simulink model "b_microCHP_constant"  (Simulink 7.6)
settings: Solver=ode45  StartTime=0  StopTime=10000000  RelTol=1e-3
undefined symbols (not defined in the file): carmen
settings Model: Creator=Sebastian  LastModifiedBy=fabian.ille  SimulationMode=accelerator
settings OptimizationCC: InitFltsAndDblsToZero=on
settings DebuggingCC: StrictBusMsg=Warning
settings SFSimCC: SimParseCustomCode=off

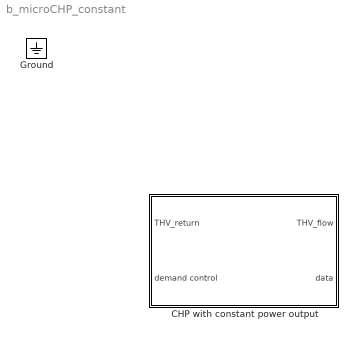
== system b_microCHP_constant ==
  CHP with constant power output : Subsystem  mask{P_th=11520, P_el=5500, P_fuel=22030, T_flow_setpoint=80, T_return_max=75}
      mask prompts: P_th "Nominal heating power [W] - at T_flow_out of 60°C"; P_el "Electrical power [W]"; P_fuel "Fuel power [W]"; T_flow_setpoint "T_flow_setpoint [°C] - Setpoint temperature of thermostat"; T_return_max "T_return_max [°C] - safety shutdown temperature"
      mask help:
      | This block is based on characteristic curves calculating heating capacity and representing a thermostat-controlled three-way mixer valve situated in the inlet flow of a gas driven micro-CHP called "Dachs" by Senertec. External mass flow rate, outlet flow temperature and heating power factor depend on inlet return temperature and are calculated by 1-D lookup-tables based on measured data.
      | The scaling is based on a heating power of 12.52 kW, an electrical power of 5.5 kW, a fuel power of 22,03 kW and a maximum external mass flow rate of 0.14 kg/s.
      | Mass flow rate and thermal inertia are linearly resized according to the inputed nominal heating power.
      mask Help: eval('filetest (''manual.htm#electric_heating'')')
      mask Display: plot(0,0,100,100,[50,50,60,40,50],[55,40,70,60,90],[59,50],[48,40])
  Ground : Ground  IOType=siggen

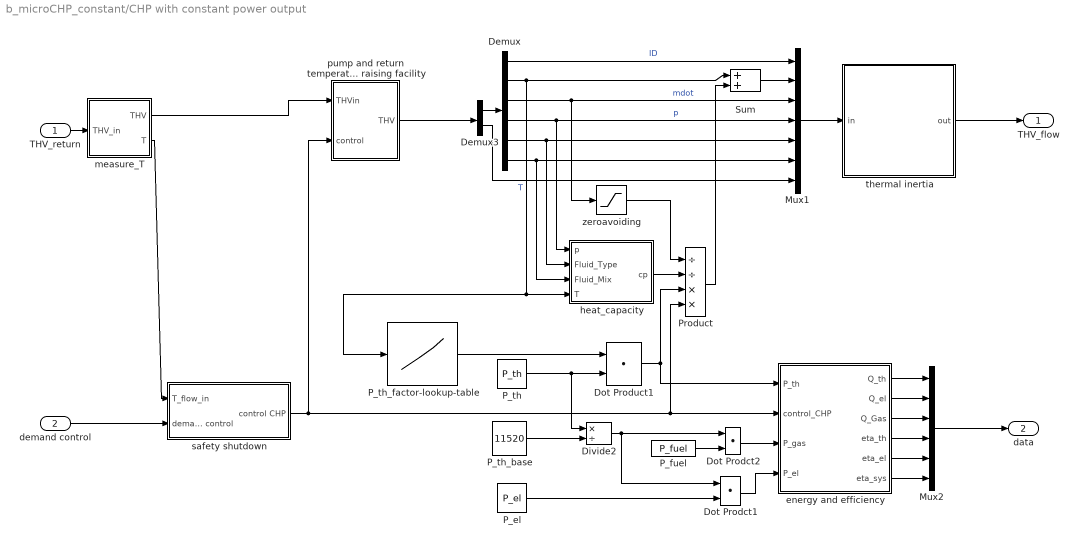
== system b_microCHP_constant/CHP with constant power output ==
  THV_return : Inport
  demand control : Inport  Port=2
  Demux : Demux  Outputs=[1 1 1 1 1 1]
  Demux3 : Demux  Outputs=[6 14]
  Divide2 : Product  Inputs=*/
  Dot Prodct1 : DotProduct  InputSameDT=on  OutDataTypeStr=Inherit: Inherit via internal rule
  Dot Prodct2 : DotProduct  InputSameDT=on  OutDataTypeStr=Inherit: Inherit via internal rule
  Dot Product1 : DotProduct  InputSameDT=on  OutDataTypeStr=Inherit: Inherit via internal rule
  Mux1 : Mux  Inputs=[1 1 1 1 1 1 14]
  Mux2 : Mux  Inputs=6
  P_el : Constant  Value=P_el
  P_fuel : Constant  Value=P_fuel
  P_th : Constant  Value=P_th
  P_th_base : Constant  Value=11520
  P_th_factor-lookup-table : Lookup_n-D  NumberOfTableDimensions=1  BreakpointsForDimension1=[45,50,60,65,74]  BreakpointsForDimension2=[44,80]  BreakpointsForDimension3=[1:2]  BreakpointsForDimension4=[1:2]  Table=[1.09 1.06 1 0.98 0.94]  InputSameDT=on
  Product : Product  Inputs=//**  SaturateOnIntegerOverflow=on  RndMeth=Zero  InputSameDT=on  OutDataTypeStr=Inherit: Same as first input
  Sum : Sum  SaturateOnIntegerOverflow=on  InputSameDT=on  OutDataTypeStr=Inherit: Same as first input
  energy and efficiency : Subsystem
  heat_capacity : Subsystem
      mask Type: heat capacity
      mask Description:
      | Calculates the  heat_capacity of fluids [J/(kg*K)].
      | Calls calls the function "hcap" in the CARNOT library "carlib".
      | Definition of the fluid types
      | fluid-ID  material           remarks on fluid mix
      | 1           water              vapourcontent in the 2-phase region
      | 2           air                   is (kg water) / (kg air)
      | 3           cotton oil
      | 4           silicone oil
      | 5           water-glycol    gives the volume partition [0..1] of glycol
      mask Help: eval('htmlhelp (''chap_4_2h.htm#heat_capacity'')')
  measure_T : Subsystem  mask(temperature measurement sensor){tc=10, t0=25}
      mask prompts: tc "time constant of sensor [s]"; t0 "initial temperature [degree centigrade]"
      mask help: Measurement sensor for temperatures with first-oder hold. Temperature is in degree centigrade.
      mask init:
      | tc = 1/max(tc, 0.001);
      mask Help: eval('man (''measure_T'')')
      mask Display: plot(-18,0,30,20,[0 20],[0 0],[10 10 8 8 12 12 10],[0 8 8 17 17 8 8],[10 10 9 9 11 11 10 9],[15 10 10 9 9 10 9 10])
  pump and return temperature raising facility : Subsystem  mask( Pump and return temperature raising facility){fluid_id=water, mix=0, dia=0.02, power=100, p0=3e5}
      mask prompts: fluid_id "fluid"; mix "percentage of fluid mix [0..1]"; dia "diameter at in- and outlet [m]"; power "electric power consumption [W]"; p0 "system pressure [Pa]"
      mask help:
      | In this modul a pump and a return temperature raising facility are modelled by two lookup-tables. They are based on measured data.
      |
      | The mass flow-lookup table gives out the mass flow (outside of CHP) depending on the return flow temperature T_return (outside of CHP). The return flow temperature (inside of CHP) is kept on 74°C by means of a thermostatic mixing valve.
      |
      | The T_flow-lookup table gives out the flow temperature T_flow depending on the return flow temperature (outside of CHP).
      |
      | The mass flow (outside of CHP) varies by means of multiplication with a factor f_flowSetpoint depending on the flow setpoint temperature T_flowSetpoint.
      | f_flowSetpoint is calculated according to the following formula:
      | (T_flow-T_return)/(T_flowSetpoint-T_return).
      |
      | The mass flow (outside of CHP) depends also on the nominal heating power P_heating and is therefor multiplied with a factor f_power.
      | f_power is calculated according to the following formula: P_heating/11520.
      mask init:
      | mix = min(1, max(0, mix));
      | dia = max(0.001, dia);
      | p0 = max(p0, 1e5);
      mask Help: eval('htmlhelp (''chap_4_2p.htm#pump_const'')')
      mask StyleString: popup(water|air|cotton_oil|silicone_oil|water_glycol_mix),edit,edit,edit,edit
      mask Display: plot(0,0,100,100,[40,70,40,30,30,40,60,70,70,60,40],[70,50,30,40,60,70,70,60,40,30,30])
  safety shutdown : Subsystem
      mask Type: control of safety shutdown
      mask Description:
      | CHP ON: T_return < T_return_max
      | CHP OFF: T_return > T_return_max
      mask Display: plot(-30,0,150,100,[70,100,40,10,70,70,10,10],[50,80,80,50,50,20,20,50],[100,70],[50,20],[20,50,50,20,20],[40,40,30,30,40],[62,62,62,61,59,58,58,60],[42,41,39,38,38,40,42,43],[61,62,62,61,60,59,58,58,58,59],[32,31,30,28,27,28,28,30,31,32])
  thermal inertia : Subsystem  LoadFcn=carmen('call');  mask(simple water storage){vol=0.00175*P_th/1000+ 0.0021, d=0.1, stand=standing cylinder, cond=1, uloss=1, tini=25, nodes=3, mpts=1, T_amb=15}
      mask prompts: vol "volume [m³]"; d "diameter [m]"; stand "position"; cond "axial heat conductivity [W/(m*K)]"; uloss "heat loss coefficient [W/(m²*K)]"; tini "initial temperature [degree centigrade]"; nodes "number of nodes"; mpts "number of measurement points (>= 3)  (first is at bottom)"; T_amb "ambient temperature"
      mask help: multinode water storage
      mask init:
      | vol = max(vol, 0.001);
      | d = max(d, 0.001);
      | stand = stand-1;
      | nodes = max(nodes, 1);
      | mpts = max(mpts, 3);
      mask Help: eval('htmlhelp (''chap_4_2s.htm#storage'')')
      mask StyleString: edit,edit,popup(lying cylinder|standing cylinder),edit,edit,edit,edit,edit,edit
      mask Display: plot(0,0,100,110,[40,40,47,53,60,60,53,47,40],[80,40,30,30,40,80,90,90,80],[40,35],[77,77],[64,60],[77,77],[40,35],[42,42],[64,60],[42,42])
  zeroavoiding : Saturate  UpperLimit=inf  LowerLimit=1e-5
  THV_flow : Outport  InitialOutput=0
  data : Outport  Port=2  InitialOutput=0
  wires:
  Demux/4 -> Mux1/4, heat_capacity/1(p)  "p"
  Demux/1 -> Mux1/1  "ID"
  Demux/5 -> heat_capacity/2(Fluid_Type), Mux1/5
  Demux/6 -> heat_capacity/3(Fluid_Mix), Mux1/6
  heat_capacity/1(cp) -> Product/2
  Demux/3 -> Mux1/3, zeroavoiding/1  "mdot"
  zeroavoiding/1 -> Product/1
  Sum/1 -> Mux1/2
  Demux3/1 -> Demux/1
  Demux3/2 -> Mux1/7
  Mux1/1 -> thermal inertia/1(in)
  thermal inertia/1(out) -> THV_flow/1
  P_th_factor-lookup-table/1 -> Dot Product1/1
  P_th/1 -> Dot Product1/2, Divide2/1
  THV_return/1 -> measure_T/1(THV_in)
  pump and return temperature raising facility/1(THV) -> Demux3/1
  Product/1 -> Sum/2
  Demux/2 -> Sum/1, heat_capacity/4(T), P_th_factor-lookup-table/1  "T"
  measure_T/2(T) -> safety shutdown/1(T_flow_in)
  Dot Product1/1 -> Product/3, energy and efficiency/1(P_th)
  safety shutdown/1(control CHP) -> Product/4, energy and efficiency/2(control_CHP), pump and return temperature raising facility/2(control)
  demand control/1 -> safety shutdown/2(demand control)
  P_th_base/1 -> Divide2/2
  P_fuel/1 -> Dot Prodct2/2
  Dot Prodct1/1 -> energy and efficiency/4(P_el)
  P_el/1 -> Dot Prodct1/2
  Divide2/1 -> Dot Prodct2/1, Dot Prodct1/1
  Dot Prodct2/1 -> energy and efficiency/3(P_gas)
  measure_T/1(THV) -> pump and return temperature raising facility/1(THVin)
  energy and efficiency/1(Q_th) -> Mux2/1
  energy and efficiency/2(Q_el) -> Mux2/2
  energy and efficiency/3(Q_Gas) -> Mux2/3
  energy and efficiency/4(eta_th) -> Mux2/4
  energy and efficiency/5(eta_el) -> Mux2/5
  energy and efficiency/6(eta_sys) -> Mux2/6
  Mux2/1 -> data/1

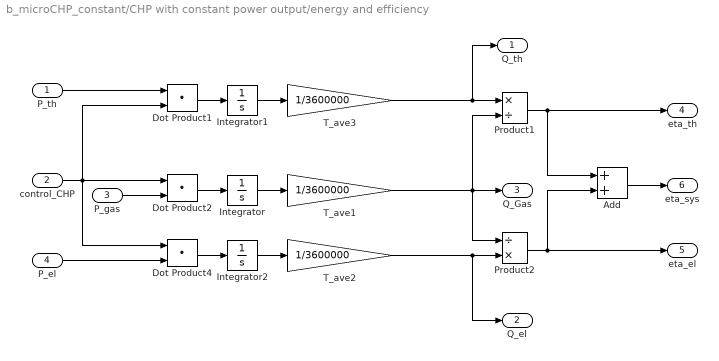
== system b_microCHP_constant/CHP with constant power output/energy and efficiency ==
  P_th : Inport
  control_CHP : Inport  Port=2
  P_gas : Inport  Port=3
  P_el : Inport  Port=4
  Add : Sum
  Dot Product1 : DotProduct  InputSameDT=on  OutDataTypeStr=Inherit: Inherit via internal rule
  Dot Product2 : DotProduct  InputSameDT=on  OutDataTypeStr=Inherit: Inherit via internal rule
  Dot Product4 : DotProduct  InputSameDT=on  OutDataTypeStr=Inherit: Inherit via internal rule
  Integrator : Integrator
  Integrator1 : Integrator
  Integrator2 : Integrator
  Product1 : Product  Inputs=*/  SaturateOnIntegerOverflow=on  RndMeth=Zero  InputSameDT=on  OutDataTypeStr=Inherit: Same as first input
  Product2 : Product  Inputs=/*  SaturateOnIntegerOverflow=on  RndMeth=Zero  InputSameDT=on  OutDataTypeStr=Inherit: Same as first input
  T_ave1 : Gain  Gain=1/3600000  SaturateOnIntegerOverflow=on  OutDataTypeStr=Inherit: Same as input  ParamDataTypeStr=Inherit: Same as input
  T_ave2 : Gain  Gain=1/3600000  SaturateOnIntegerOverflow=on  OutDataTypeStr=Inherit: Same as input  ParamDataTypeStr=Inherit: Same as input
  T_ave3 : Gain  Gain=1/3600000  SaturateOnIntegerOverflow=on  OutDataTypeStr=Inherit: Same as input  ParamDataTypeStr=Inherit: Same as input
  Q_th : Outport  InitialOutput=0
  Q_el : Outport  Port=2  InitialOutput=0
  Q_Gas : Outport  Port=3  InitialOutput=0
  eta_th : Outport  Port=4  InitialOutput=0
  eta_el : Outport  Port=5  InitialOutput=0
  eta_sys : Outport  Port=6  InitialOutput=0
  wires:
  P_gas/1 -> Dot Product2/2
  Integrator/1 -> T_ave1/1
  Integrator2/1 -> T_ave2/1
  P_el/1 -> Dot Product4/2
  Product2/1 -> eta_el/1, Add/2
  Dot Product4/1 -> Integrator2/1
  Dot Product2/1 -> Integrator/1
  control_CHP/1 -> Dot Product2/1, Dot Product4/1, Dot Product1/2
  T_ave1/1 -> Product2/1, Q_Gas/1, Product1/2
  T_ave2/1 -> Product2/2, Q_el/1
  Dot Product1/1 -> Integrator1/1
  P_th/1 -> Dot Product1/1
  Integrator1/1 -> T_ave3/1
  T_ave3/1 -> Product1/1, Q_th/1
  Product1/1 -> Add/1, eta_th/1
  Add/1 -> eta_sys/1

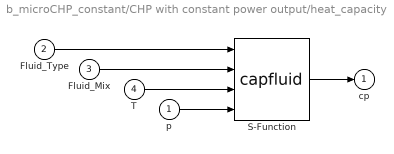
== system b_microCHP_constant/CHP with constant power output/heat_capacity ==
  p : Inport
  Fluid_Type : Inport  Port=2
  Fluid_Mix : Inport  Port=3
  T : Inport  Port=4
  S-Function : S-Function  FunctionName=capfluid  EnableBusSupport=off
      mask Description:
      | Calculates the heat_capacity
      | 
      | INPUT VECTORS:
      | fluid type [1..5]
      | fluid mix
      | temperature [°C]
      | pressure [Pa]
      | 
      | OUTPUT VECTOR:
      | heat_capacity [J/(kg K)]
  cp : Outport  InitialOutput=0
  wires:
  p/1 -> S-Function/4
  T/1 -> S-Function/3
  Fluid_Mix/1 -> S-Function/2
  Fluid_Type/1 -> S-Function/1
  S-Function/1 -> cp/1

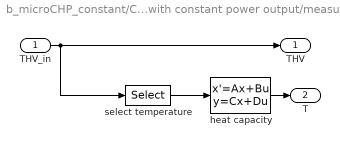
== system b_microCHP_constant/CHP with constant power output/measure_T ==
  THV_in : Inport
  heat capacity : StateSpace  A=-tc  B=tc  D=0  X0=t0
  select temperature : Selector  InputPortWidth=20  IndexOptions=Index vector (dialog)  Indices=[2]  OutputSizes=1
  THV : Outport  InitialOutput=0
  T : Outport  Port=2  InitialOutput=0
  wires:
  THV_in/1 -> select temperature/1, THV/1
  select temperature/1 -> heat capacity/1
  heat capacity/1 -> T/1

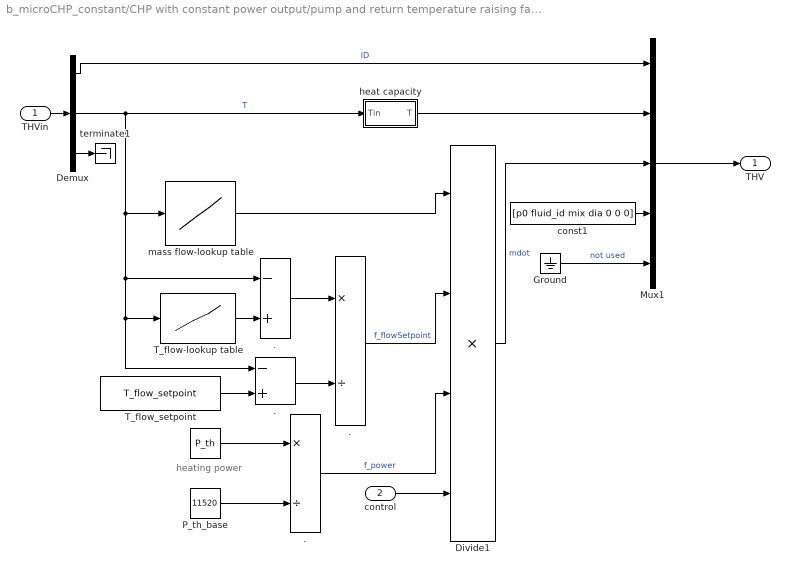
== system b_microCHP_constant/CHP with constant power output/pump and return temperature raising facility ==
  note: heating power
  THVin : Inport
  control : Inport  Port=2
  " " : Constant  Value=P_th
  " ." : Product  Inputs=*/
  " .  " : Sum  Inputs=-+
  . : Sum  Inputs=-+
  ". " : Product  Inputs=*/
  Demux : Demux  Outputs=[1 1 18]
  Divide1 : Product  Inputs=****
  Ground : Ground
  Mux1 : Mux  Inputs=[1 1 1 7 10]
  P_th_base : Constant  Value=11520
  T_flow-lookup table : Lookup_n-D  NumberOfTableDimensions=1  BreakpointsForDimension1=[45,50,60,65,74]  BreakpointsForDimension2=[44,80]  BreakpointsForDimension3=[1:2]  BreakpointsForDimension4=[1:2]  Table=[78.5 79.65 81 84.18 92.47]  InputSameDT=on
  T_flow_setpoint : Constant  Value=T_flow_setpoint
  const1 : Constant  Value=[p0 fluid_id mix dia 0 0 0]
  heat capacity : Subsystem  mask{NTU=3.3}
      mask prompts: NTU "NTU (k*A/(m*cp))"
  mass flow-lookup table : Lookup_n-D  NumberOfTableDimensions=1  BreakpointsForDimension1=[45,50,60,65,74]  BreakpointsForDimension2=[44,80]  BreakpointsForDimension3=[1:2]  BreakpointsForDimension4=[1:2]  Table=[0.09 0.1 0.129 0.139 0.140]  InputSameDT=on
  terminate1 : Terminator
  THV : Outport  InitialOutput=0
  wires:
  Ground/1 -> Mux1/5  "not used"
  Demux/1 -> Mux1/1  "ID"
  Mux1/1 -> THV/1
  Demux/2 -> heat capacity/1(Tin), mass flow-lookup table/1, ./1, T_flow-lookup table/1, " .  "/1  "T"
  heat capacity/1(T) -> Mux1/2
  Demux/3 -> terminate1/1
  const1/1 -> Mux1/4
  THVin/1 -> Demux/1
  " "/1 -> " ."/1
  mass flow-lookup table/1 -> Divide1/1
  Divide1/1 -> Mux1/3  "mdot"
  ./1 -> ". "/1
  " .  "/1 -> ". "/2
  T_flow_setpoint/1 -> " .  "/2
  T_flow-lookup table/1 -> ./2
  P_th_base/1 -> " ."/2
  ". "/1 -> Divide1/2  "f_flowSetpoint"
  " ."/1 -> Divide1/3  "f_power"
  control/1 -> Divide1/4

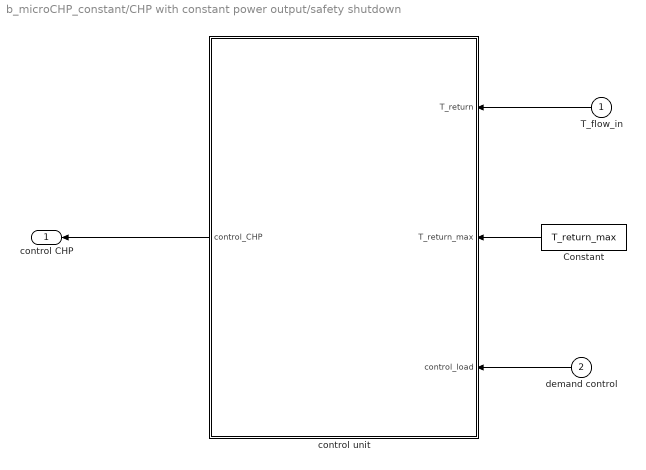
== system b_microCHP_constant/CHP with constant power output/safety shutdown ==
  T_flow_in : Inport
  demand control : Inport  Port=2
  Constant : Constant  Value=T_return_max
  control unit : Stateflow chart  TreatAsAtomicUnit=on
  control CHP : Outport
  wires:
  control unit/1(control_CHP) -> control CHP/1
  Constant/1 -> control unit/2(T_return_max)
  T_flow_in/1 -> control unit/1(T_return)
  demand control/1 -> control unit/3(control_load)

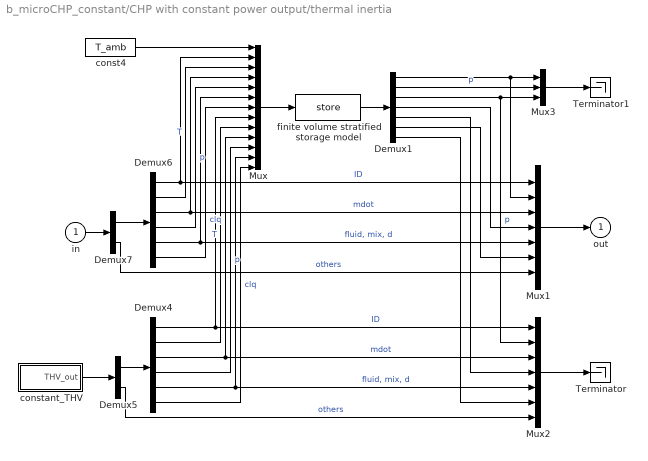
== system b_microCHP_constant/CHP with constant power output/thermal inertia ==
  in : Inport
  Demux1 : Demux  Outputs=[1 mpts-2 1 1 1 3 3]
  Demux4 : Demux  Outputs=[1 1 1 1 3 3]
  Demux5 : Demux  Outputs=[10 -1]
  Demux6 : Demux  Outputs=[1 1 1 1 3 3]
  Demux7 : Demux  Outputs=[10 -1]
  Mux : Mux  Inputs=13
  Mux1 : Mux  Inputs=7
  Mux2 : Mux  Inputs=7
  Mux3 : Mux  Inputs=3
  Terminator : Terminator
  Terminator1 : Terminator
  const4 : Constant  Value=T_amb
  constant_THV : Subsystem  mask(constant THV){t=20, mdot=0, p=2e5, fluid=water, mix=0, dia=0.02}
      mask prompts: t "temperature [degree centigrade]"; mdot "massflow [kg/s]"; p "pressure [Pa]"; mix "fluid mixture [0..1]"; dia "diameter [m]"
      mask help: Create a constant Thermo-Hydraulic-Vector.
      mask init:
      | mix = min(1, max(0, mix));
      | dia = max(dia, 0.001);
      mask Help: eval('man (''constant_THV'')')
      mask StyleString: edit,edit,edit,popup(water|air|cotton_oil|silicone_oil|water_glycol_mix|tyfocor_LS),edit,edit
  finite volume stratified storage model : S-Function  FunctionName=store  Parameters=vol, d, stand, uloss, cond, tini, nodes, mpts  EnableBusSupport=off
  out : Outport  InitialOutput=0
  wires:
  Demux1/7 -> Mux2/6
  Demux5/2 -> Mux2/7  "others"
  Demux1/6 -> Mux1/6
  Demux1/5 -> Mux2/4
  Demux4/2 -> Mux/9  "T"
  Mux2/1 -> Terminator/1
  Demux4/4 -> Mux/11  "p"
  Demux4/6 -> Mux/13  "clq"
  Demux5/1 -> Demux4/1
  Demux4/1 -> Mux/8, Mux2/1  "ID"
  Demux4/3 -> Mux/10, Mux2/3  "mdot"
  Demux4/5 -> Mux/12, Mux2/5  "fluid, mix, d"
  constant_THV/1(THV_out) -> Demux5/1
  Demux7/2 -> Mux1/7  "others"
  Demux1/3 -> Mux3/3, Mux2/2  "p"
  Demux1/2 -> Mux3/2  "p"
  Demux1/1 -> Mux3/1, Mux1/2
  Mux3/1 -> Terminator1/1
  Demux6/6 -> Mux/7  "clq"
  Demux7/1 -> Demux6/1
  in/1 -> Demux7/1
  Demux1/4 -> Mux1/4
  Mux/1 -> finite volume stratified storage model/1
  const4/1 -> Mux/1
  Mux1/1 -> out/1
  Demux6/1 -> Mux1/1, Mux/2  "ID"
  Demux6/2 -> Mux/3  "T"
  Demux6/3 -> Mux/4, Mux1/3  "mdot"
  Demux6/4 -> Mux/5  "p"
  finite volume stratified storage model/1 -> Demux1/1
  Demux6/5 -> Mux/6, Mux1/5  "fluid, mix, d"

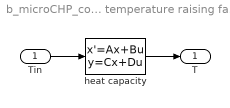
== system b_microCHP_constant/CHP with constant power output/pump and return temperature raising facility/heat capacity ==
  Tin : Inport
  heat capacity : StateSpace  A=-NTU  B=NTU  D=0  X0=80
  T : Outport
  wires:
  heat capacity/1 -> T/1
  Tin/1 -> heat capacity/1

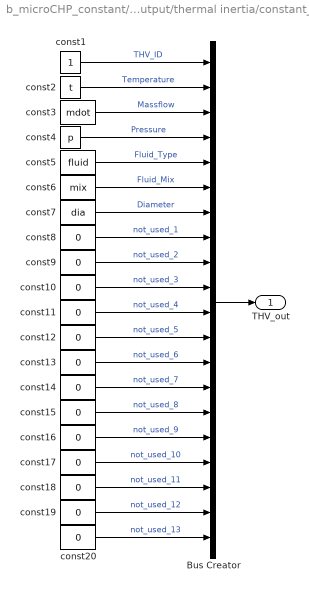
== system b_microCHP_constant/CHP with constant power output/thermal inertia/constant_THV ==
  Bus Creator : BusCreator  Inputs=20
  const1 : Constant
  const{8..20} (13 alike) : Constant  Value=0
  const2 : Constant  Value=t
  const3 : Constant  Value=mdot
  const4 : Constant  Value=p
  const5 : Constant  Value=fluid
  const6 : Constant  Value=mix
  const7 : Constant  Value=dia
  THV_out : Outport  InitialOutput=0
  wires:
  const20/1 -> Bus Creator/20  "not_used_13"
  const19/1 -> Bus Creator/19  "not_used_12"
  const18/1 -> Bus Creator/18  "not_used_11"
  const17/1 -> Bus Creator/17  "not_used_10"
  const16/1 -> Bus Creator/16  "not_used_9"
  const15/1 -> Bus Creator/15  "not_used_8"
  const14/1 -> Bus Creator/14  "not_used_7"
  const13/1 -> Bus Creator/13  "not_used_6"
  const12/1 -> Bus Creator/12  "not_used_5"
  const11/1 -> Bus Creator/11  "not_used_4"
  const10/1 -> Bus Creator/10  "not_used_3"
  const9/1 -> Bus Creator/9  "not_used_2"
  const8/1 -> Bus Creator/8  "not_used_1"
  const7/1 -> Bus Creator/7  "Diameter"
  const6/1 -> Bus Creator/6  "Fluid_Mix"
  const5/1 -> Bus Creator/5  "Fluid_Type"
  const4/1 -> Bus Creator/4  "Pressure"
  const3/1 -> Bus Creator/3  "Massflow"
  const2/1 -> Bus Creator/2  "Temperature"
  const1/1 -> Bus Creator/1  "THV_ID"
  Bus Creator/1 -> THV_out/1

== stateflow chart CHP with constant power output/safety shutdown/control unit ==
  state OFF/
    entry:control_CHP=0;
  state ON/
    entry:control_CHP=1;
  (junction 5) -> OFF [order 2]
  OFF -> ON : [T_return<T_return_max&control_load==1]
  ON -> OFF : [T_return>T_return_max |control_load==0]
  (junction 5) -> ON [order 1] : [T_return<T_return_max & control_load==1]
  (default) -> (junction 5)
  data: T_return input double; T_return_max input double =78; control_CHP output double =78; control_load input double
